simulink model "DC_Motor_Model"  (R2018a)
settings: Solver=VariableStepAuto  StartTime=0.0  StopTime=10.0  RelTol=1e-3
values from neighbouring files (symbols this model uses):
  b = 0.1    [DC_Motormfile.m]
  JM = 0.4    [DC_Motormfile.m]
  KE = 0.12    [DC_Motormfile.m]    (also in pid.m)
  KT = 0.25    [DC_Motormfile.m]    (also in pid.m)
  L = 493*10^-9    (= 4.93e-07)    [DC_Motormfile.m]    (also in pid.m)
  R = 5.3*10^-3    (= 0.0053)    [DC_Motormfile.m]    (also in pid.m)
settings Model: Creator=MAFAZ  LastModifiedBy=MAFAZ

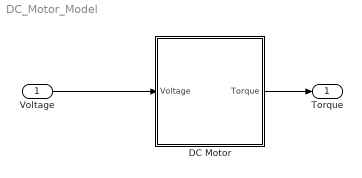
== system DC_Motor_Model ==
  Voltage : Inport
  DC Motor : Subsystem
  Torque : Outport
  wires:
  Voltage/1 -> DC Motor/1(Voltage)
  DC Motor/1(Torque) -> Torque/1

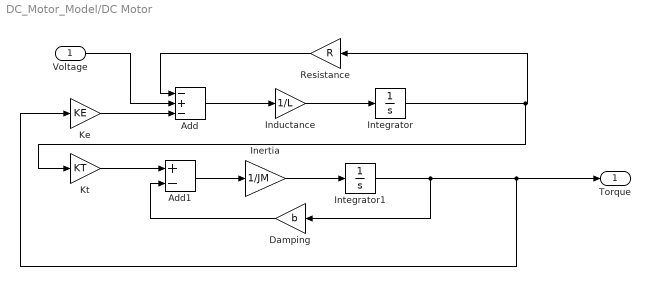
== system DC_Motor_Model/DC Motor ==
  Voltage : Inport
  Add : Sum  Inputs=-+-
  Add1 : Sum  Inputs=+-
  Damping : Gain  Gain=b
  Inductance : Gain  Gain=1/L
  Inertia : Gain  Gain=1/JM
  Integrator : Integrator
  Integrator1 : Integrator
  Ke : Gain  Gain=KE
  Kt : Gain  Gain=KT
  Resistance : Gain  Gain=R
  Torque : Outport
  wires:
  Damping/1 -> Add1/2
  Add1/1 -> Inertia/1
  Integrator/1 -> Kt/1, Resistance/1
  Inertia/1 -> Integrator1/1
  Ke/1 -> Add/3
  Add/1 -> Inductance/1
  Voltage/1 -> Add/2
  Inductance/1 -> Integrator/1
  Integrator1/1 -> Damping/1, Torque/1, Ke/1
  Kt/1 -> Add1/1
  Resistance/1 -> Add/1
